simulink model "awe_dt"  (R2024b)
settings: Solver=VariableStepAuto  StartTime=0.0  StopTime=0.001  RelTol=1e-3
model workspace (MAT data in the model file):
  A = Simulink.Parameter
  A.Value = 0.03
  A.Complexity = 'real'
  A.Dimensions = [1 1]
  A.DataType = 'double'
  A.DocUnits = 'm'
  I = Simulink.Parameter
  I.Value = Simulink.data.Expression
  I.Value.ExpressionString = "linspace(0,150,200)"
  I.Complexity = 'real'
  I.Dimensions = -1
  I.DataType = 'auto'
  I.DocUnits = 'A'
  P_an = Simulink.Parameter
  P_an.Value = 1
  P_an.Complexity = 'real'
  P_an.Dimensions = [1 1]
  P_an.DataType = 'auto'
  P_an.DocUnits = 'bar'
  P_cat = Simulink.Parameter
  P_cat.Value = 1
  P_cat.Complexity = 'real'
  P_cat.Dimensions = [1 1]
  P_cat.DataType = 'auto'
  P_cat.DocUnits = 'bar'
  T = Simulink.Parameter
  T.Value = Simulink.data.Expression
  T.Value.ExpressionString = "(linspace(273.15,353.15,8))'"
  T.Complexity = 'real'
  T.Dimensions = -1
  T.DataType = 'auto'
  T.DocUnits = 'K'
  Voltage = Simulink.Signal
  Voltage.Dimensions = -1
  Voltage.DimensionsMode = 'auto'
  Voltage.Complexity = 'auto'
  Voltage.SampleTime = -1
  Voltage.SamplingMode = 'auto'
  Voltage.DataType = 'auto'
  molality_koh = Simulink.Parameter
  molality_koh.Value = 5.94
  molality_koh.Complexity = 'real'
  molality_koh.Dimensions = [1 1]
  molality_koh.DataType = 'auto'
  molality_koh.DocUnits = 'mol/kg'
settings Model: Creator=vr231  LastModifiedBy=jnana

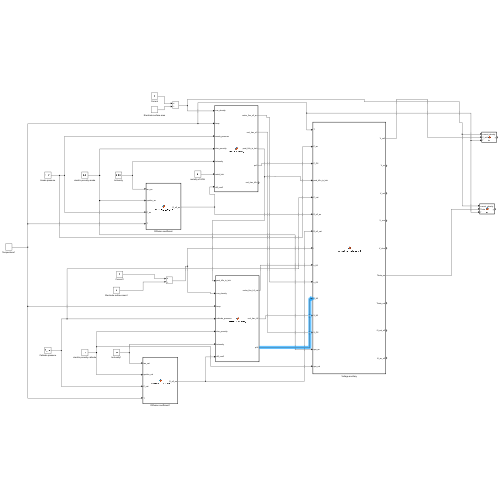
[thumbnail: Simulink's stored preview of the top-level diagram]
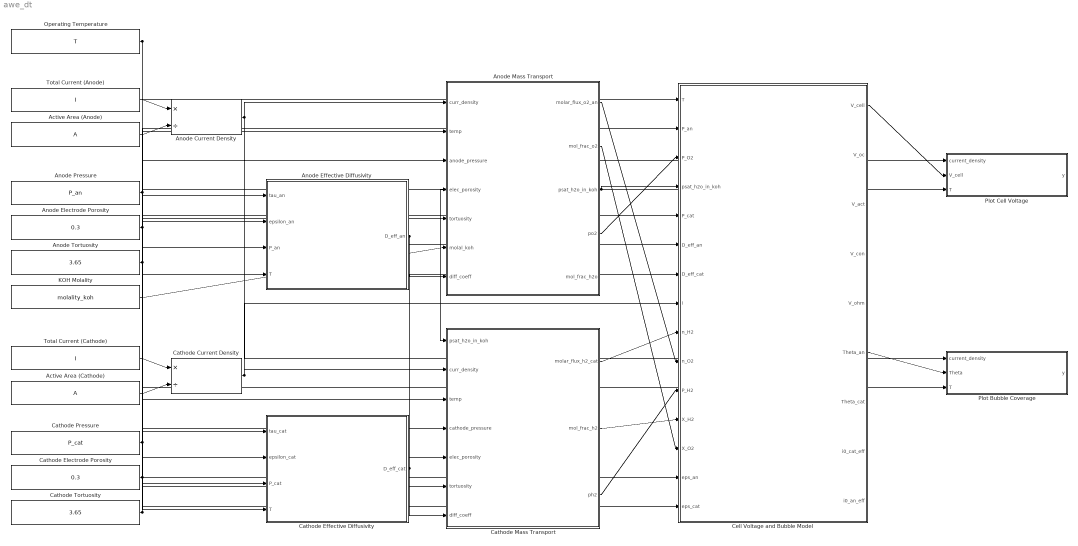
== system awe_dt ==
  Anode Pressure : Constant  Value=P_an
  Cathode Pressure : Constant  Value=P_cat
  Total Current (Anode) : Constant  Value=I
  Total Current (Cathode) : Constant  Value=I
  Anode Effective Diffusivity : MATLAB Function  TreatAsAtomicUnit=on
  Cathode Effective Diffusivity : MATLAB Function  TreatAsAtomicUnit=on
  Anode Current Density : Product  Inputs=*/
  Cathode Current Density : Product  Inputs=*/
  Active Area (Anode) : Constant  Value=A
  Active Area (Cathode) : Constant  Value=A
  Anode Mass Transport : MATLAB Function  TreatAsAtomicUnit=on
  Cathode Mass Transport : MATLAB Function  TreatAsAtomicUnit=on
  Plot Bubble Coverage : MATLAB Function  TreatAsAtomicUnit=on
  Plot Cell Voltage : MATLAB Function  TreatAsAtomicUnit=on
  Operating Temperature : Constant  Value=T
  Cell Voltage and Bubble Model : MATLAB Function  TreatAsAtomicUnit=on
  Anode Electrode Porosity : Constant  Value=0.3
  Cathode Electrode Porosity : Constant  Value=0.3
  KOH Molality : Constant  Value=molality_koh
  Anode Tortuosity : Constant  Value=3.65
  Cathode Tortuosity : Constant  Value=3.65
  wires:
  KOH Molality/1 -> Anode Mass Transport/6(molal_koh)
  Operating Temperature/1 -> Cathode Effective Diffusivity/4(T), Cathode Mass Transport/3(temp), Plot Bubble Coverage/3(T), Plot Cell Voltage/3(T), Cell Voltage and Bubble Model/1(T), Anode Mass Transport/2(temp), Anode Effective Diffusivity/4(T)
  Anode Pressure/1 -> Cell Voltage and Bubble Model/2(P_an), Anode Mass Transport/3(anode_pressure), Anode Effective Diffusivity/3(P_an)
  Total Current (Anode)/1 -> Anode Current Density/1
  Active Area (Anode)/1 -> Anode Current Density/2
  Anode Effective Diffusivity/1(D_eff_an) -> Anode Mass Transport/7(diff_coeff), Cell Voltage and Bubble Model/6(D_eff_an)
  Anode Tortuosity/1 -> Anode Effective Diffusivity/1(tau_an), Anode Mass Transport/5(tortuosity)
  Anode Electrode Porosity/1 -> Cell Voltage and Bubble Model/14(eps_an), Anode Effective Diffusivity/2(epsilon_an), Anode Mass Transport/4(elec_porosity)
  Cathode Effective Diffusivity/1(D_eff_cat) -> Cell Voltage and Bubble Model/7(D_eff_cat), Cathode Mass Transport/7(diff_coeff)
  Cathode Pressure/1 -> Cell Voltage and Bubble Model/5(P_cat), Cathode Mass Transport/4(cathode_pressure), Cathode Effective Diffusivity/3(P_cat)
  Cathode Electrode Porosity/1 -> Cell Voltage and Bubble Model/15(eps_cat), Cathode Mass Transport/5(elec_porosity), Cathode Effective Diffusivity/2(epsilon_cat)
  Active Area (Cathode)/1 -> Cathode Current Density/2
  Cathode Current Density/1 -> Cathode Mass Transport/2(curr_density), Cell Voltage and Bubble Model/8(i)
  Total Current (Cathode)/1 -> Cathode Current Density/1
  Cathode Tortuosity/1 -> Cathode Mass Transport/6(tortuosity), Cathode Effective Diffusivity/1(tau_cat)
  Anode Mass Transport/3(psat_h2o_in_koh) -> Cell Voltage and Bubble Model/4(psat_h2o_in_koh), Cathode Mass Transport/1(psat_h2o_in_koh)
  Anode Mass Transport/1(molar_flux_o2_an) -> Cell Voltage and Bubble Model/10(n_O2)
  Cathode Mass Transport/2(mol_frac_h2) -> Cell Voltage and Bubble Model/12(X_H2)
  Cathode Mass Transport/1(molar_flux_h2_cat) -> Cell Voltage and Bubble Model/9(n_H2)
  Anode Mass Transport/2(mol_frac_o2) -> Cell Voltage and Bubble Model/13(X_O2)
  Cell Voltage and Bubble Model/1(V_cell) -> Plot Cell Voltage/2(V_cell)
  Cathode Mass Transport/3(ph2) -> Cell Voltage and Bubble Model/11(P_H2)
  Cell Voltage and Bubble Model/6(Theta_an) -> Plot Bubble Coverage/2(Theta)
  Anode Current Density/1 -> Plot Bubble Coverage/1(current_density), Plot Cell Voltage/1(current_density), Anode Mass Transport/1(curr_density)
  Anode Mass Transport/4(po2) -> Cell Voltage and Bubble Model/3(P_O2)

== matlab function awe_dt/Plot Bubble Coverage ==
  data: current_density input; y output; Theta input; T input
function y = fcn(current_density, Theta, T)
%#codegen
  % Define graphics functions as extrinsic
  coder.extrinsic('figure','axes','plot','xlabel','ylabel','drawnow','hold','grid','isvalid','cla','box','legend','sprintf');
  
  persistent hFig hAx plot_done
  
  % --- FIGURE SETUP ---
  if isempty(hFig)
      hFig = figure('Name','Theta vs Current','NumberTitle','off');
      hAx  = axes('Parent',hFig);
      xlabel(hAx,'Current Density (A/m^2)');  
      ylabel(hAx,'Bubble Coverage (Theta)');
      grid(hAx, 'on'); box(hAx, 'on'); hold(hAx, 'on');
      plot_done = [];
  end
  
  if ~isvalid(hFig)
      hFig = figure('Name','Theta vs Current','NumberTitle','off');
      hAx  = axes('Parent',hFig);
      xlabel(hAx,'Current Density (A/m^2)');  
      ylabel(hAx,'Bubble Coverage (Theta)');
      grid(hAx, 'on'); box(hAx, 'on'); hold(hAx, 'on');
      plot_done = [];
  end
  
  % --- DATA PREP (No Resizing Inputs) ---
  u_plot = double(current_density); 
  v_plot = double(Theta);           
  T_vals = double(T);            
  
  % Transpose logic for PLOTTING ONLY. 
  if size(v_plot, 2) == numel(u_plot)
      v_plot_T = v_plot.'; 
  else
      v_plot_T = v_plot;
  end
  
  % --- PLOT ---
  if isempty(plot_done)
      cla(hAx); 
      plot(hAx, u_plot, v_plot_T, '-o', 'LineWidth', 1.5, 'MarkerSize', 4);
      
      % --- LEGEND (Extrinsic Call) ---
      update_legend(hAx, T_vals);
      
      drawnow;
      plot_done = 1;
  end
  % --- OUTPUT ---
  y = Theta;
end

% --- SUB-FUNCTION (Runs in MATLAB only) ---
function update_legend(ax_handle, T_vals)
    if numel(T_vals) > 0
        labels = cell(1, numel(T_vals));
        for k = 1:numel(T_vals)
            % CHANGED: Using sprintf instead of num2str
            labels{k} = sprintf('T = %.1f K', T_vals(k));
        end
        legend(ax_handle, labels, 'Location', 'best');
    end
end

== matlab function awe_dt/Plot Cell Voltage ==
  data: current_density input; y output; V_cell input; T input
function y = fcn(current_density, V_cell, T)
%#codegen
  % Define graphics functions as extrinsic
  coder.extrinsic('figure','axes','plot','xlabel','ylabel','drawnow','hold','grid','isvalid','cla','box','legend','sprintf');
  
  persistent hFig hAx plot_done
  
  % --- FIGURE SETUP ---
  if isempty(hFig)
      hFig = figure('Name','Voltage vs Current','NumberTitle','off');
      hAx  = axes('Parent',hFig);
      xlabel(hAx,'Current Density (A/m^2)');  
      ylabel(hAx,'Cell Voltage (V)');
      grid(hAx, 'on'); box(hAx, 'on'); hold(hAx, 'on');    
      plot_done = [];
  end
  
  if ~isvalid(hFig)
      hFig = figure('Name','Voltage vs Current','NumberTitle','off');
      hAx  = axes('Parent',hFig);
      xlabel(hAx,'Current Density (A/m^2)');  
      ylabel(hAx,'Cell Voltage (V)');
      grid(hAx, 'on'); box(hAx, 'on'); hold(hAx, 'on');
      plot_done = [];
  end
  
  % --- DATA PREP (No Resizing Inputs) ---
  if isempty(plot_done)
      u_plot = double(current_density); 
      v_plot = double(V_cell);           
      T_vals = double(T);            
      
      % Transpose logic for PLOTTING ONLY. 
      % We assume u_plot is 1x201. v_plot is 8x201.
      % Plot expects 201x8.
      if size(v_plot, 2) == numel(u_plot)
          v_plot_T = v_plot.'; 
      else
          v_plot_T = v_plot;
      end
      
      % --- PLOT ---
      cla(hAx); 
      plot(hAx, u_plot, v_plot_T, 'o', 'LineWidth', 1.5, 'MarkerSize', 4);
      
      % --- LEGEND (Extrinsic Call) ---
      update_legend(hAx, T_vals);
      
      drawnow;
      plot_done = 1;
  end 
  % --- OUTPUT ---
  y = V_cell;
end

% --- SUB-FUNCTION (Runs in MATLAB only) ---
function update_legend(ax_handle, T_vals)
    if numel(T_vals) > 0
        labels = cell(1, numel(T_vals));
        for k = 1:numel(T_vals)
            % Clean formatting for Legend
            labels{k} = sprintf('T = %.1f K', T_vals(k));
        end
        legend(ax_handle, labels, 'Location', 'best');
    end
end

== matlab function awe_dt/Anode Effective Diffusivity ==
  data: tau_an input; epsilon_an input; P_an input; T input; D_eff_an output
function D_eff_an = calculate_D_eff_an( tau_an,epsilon_an,P_an,T)
    % Calculates the effective binary diffusion coefficient at the anode (D_eff_an)
    % according to equations 38-46 from Abdin et al. (2017)
    %
    % Inputs:
    %   T - Temperature [K]
    %   P_an - Anode pressure [Pa]
    %   epsilon_an - Anode porosity [dimensionless]
    %   tau_an - Anode tortuosity [dimensionless]
    %
    % Output:
    %   D_eff_an - Effective binary diffusion coefficient at anode [m^2/s]

    % Constants
    R = 8.314;               % Universal gas constant [J/(mol·K)]
    k = 1.38064852e-23;      % Boltzmann constant [J/K]
    
    % Molecular weights [kg/mol]
    M_O2 = 32e-3;
    M_H2O = 18e-3;
    
    % Molecular radii [m] (converted from Å)
    sigma_O2 = 3.467e-10;
    sigma_H2O = 2.641e-10;
    
    % Lennard-Jones potentials [K]
    epsilon_O2_k = 106.7;    % epsilon/k for O2
    epsilon_H2O_k = 809.1;   % epsilon/k for H2O
    
    % Convert Lennard-Jones potentials to Joules
    epsilon_O2 = epsilon_O2_k * k;
    epsilon_H2O = epsilon_H2O_k * k;
    
    % Mean pore radius [m] (typical value, can be adjusted)
    r = 75e-9;                % 75 nm
    
    % Calculate mean molecular radius (Eq. 44)
    sigma_O2_H2O = (sigma_O2 + sigma_H2O)/2;
    
    % Calculate Lennard-Jones energy (Eq. 46)
    epsilon_O2_H2O = sqrt(epsilon_O2 * epsilon_H2O);
    
    % Calculate reduced temperature (Eq. 45)
    tau_O2_H2O = k .* T / epsilon_O2_H2O;
    
    % Calculate dimensionless diffusion collision integral (Eq. 43)
    Omega_D = 1.06./(tau_O2_H2O.^0.156) + 0.193./exp(0.476.*tau_O2_H2O) + ...
              1.036./exp(1.53.*tau_O2_H2O) + 1.765./(3.894.*tau_O2_H2O);
    
    % Calculate effective molecular binary diffusion coefficient (Eq. 41)
    D_eff_O2_H2O = 0.00133 .* (1/M_O2 + 1/M_H2O)^0.5 .* T.^1.5 ./ ...
                  (P_an.*(10^5).* sigma_O2_H2O^2 .* Omega_D);
    
    % Calculate effective Knudsen diffusion coefficient (Eq. 40)
    D_eff_H2O_K = (4/3) * r * sqrt((8 * R .* T) / (pi * M_H2O));
    
    % Calculate effective binary diffusion coefficient at anode (Eq. 38)
    D_eff_an = ((epsilon_an ./ tau_an) .* (1./D_eff_O2_H2O + 1./D_eff_H2O_K).^-1);
end

== matlab function awe_dt/Anode Mass Transport ==
  data: curr_density input; temp input; molar_flux_o2_an output; anode_pressure input; elec_porosity input; mol_frac_o2 output; psat_h2o_in_koh output; po2 output; tortuosity input; molal_koh input; diff_coeff input; mol_frac_h2o output
function [molar_flux_o2_an, mol_frac_o2, psat_h2o_in_koh, po2, mol_frac_h2o] = anode_ancillary(curr_density, temp, anode_pressure, elec_porosity, tortuosity, molal_koh, diff_coeff)
    % Constants
    faraday_const = 96485;       % C/mol
    univ_gas_const = 8.314;       % J/(mol·K)
    len_an_to_catalyst = 0.002;   % m

    % Ensure vector orientations
    curr_density = curr_density(:).';  % Force row vector [1×m]
    temp = temp(:);                    % Force column vector [n×1]
    
    % Nested function for water vapor pressure
    function log_pw = calculate_logpw(m, T)
        term1 = -0.01508*m - 0.0016788*m.^2 + 2.25887e-5*m.^3;
        poly_m = 1 - 0.0012062*m + 5.6024e-4*m.^2 - 7.8228e-6*m.^3;
        term_T = 35.4462 - 3343.93./T - 10.9*log10(T) + 0.0041645*T;
        log_pw = term1 + poly_m.*term_T;
    end

    % 1. Calculate water vapor pressure [n×1]
    psat_h2o_in_koh = 10.^(calculate_logpw(molal_koh, temp));  % bar

    % 2. Molar oxygen flux [1×m]
    molar_flux_o2_an = curr_density ./ (4 * faraday_const);  % mol/(m²·s)

    % 3. Water mole fraction calculation [n×m]
    R = univ_gas_const;
    L = len_an_to_catalyst;
    F = faraday_const;
    P = anode_pressure * 1e5;  % Convert bar to Pa
    
    % Calculate exponent term with dimensional consistency
    exponent_term = (R * L) ./ (2 * F * P * diff_coeff) .* (curr_density .* temp);
    
    % Clamp exponent to prevent overflow
    max_exp = 700;  % exp(700) ≈ 1e304 (below realmax)
    exponent_term = min(exponent_term, max_exp);
    
    % Calculate mole fraction with safeguards
    mol_frac_h2o = (elec_porosity/tortuosity) .* exp(exponent_term);
    mol_frac_h2o = min(mol_frac_h2o, 1);  % Prevent values >1
    mol_frac_h2o = max(mol_frac_h2o, 0);  % Prevent negative values

    % 4. Oxygen mole fraction [n×m]
    mol_frac_o2 = 1 - mol_frac_h2o;

    % 5. Oxygen partial pressure [n×m]
    po2 = ((1 ./ mol_frac_h2o) - 1) .* psat_h2o_in_koh;  % bar
end

== matlab function awe_dt/Cathode Effective Diffusivity ==
  data: tau_cat input; epsilon_cat input; P_cat input; T input; D_eff_cat output
function D_eff_cat = calculate_D_eff_cat( tau_cat,epsilon_cat,P_cat,T)
    % Calculates the effective binary diffusion coefficient at the anode (D_eff_cat)
    % according to equations 38-46 from Abdin et al. (2017)
    %
    % Inputs:
    %   T - Temperature [K]
    %   P_an - Anode pressure [Pa]
    %   epsilon_an - Anode porosity [dimensionless]
    %   tau_an - Anode tortuosity [dimensionless]
    %
    % Output:
    %   D_eff_cat - Effective binary diffusion coefficient at anode [m^2/s]

    % Constants
    R = 8.314;               % Universal gas constant [J/(mol·K)]
    k = 1.38064852e-23;      % Boltzmann constant [J/K]
    
    % Molecular weights [kg/mol]
    M_O2 = 32e-3;
    M_H2O = 18e-3;
    
    % Molecular radii [m] (converted from Å)
    sigma_O2 = 3.467e-10;
    sigma_H2O = 2.641e-10;
    
    % Lennard-Jones potentials [K]
    epsilon_O2_k = 106.7;    % epsilon/k for O2
    epsilon_H2O_k = 809.1;   % epsilon/k for H2O
    
    % Convert Lennard-Jones potentials to Joules
    epsilon_O2 = epsilon_O2_k * k;
    epsilon_H2O = epsilon_H2O_k * k;
    
    % Mean pore radius [m] (typical value, can be adjusted)
    r = 75e-9;                % 75 nm
    
    % Calculate mean molecular radius (Eq. 44)
    sigma_O2_H2O = (sigma_O2 + sigma_H2O)/2;
    
    % Calculate Lennard-Jones energy (Eq. 46)
    epsilon_O2_H2O = sqrt(epsilon_O2 * epsilon_H2O);
    
    % Calculate reduced temperature (Eq. 45)
    tau_O2_H2O = k .* T / epsilon_O2_H2O;
    
    % Calculate dimensionless diffusion collision integral (Eq. 43)
    Omega_D = 1.06./(tau_O2_H2O.^0.156) + 0.193./exp(0.476.*tau_O2_H2O) + ...
              1.036./exp(1.53.*tau_O2_H2O) + 1.765./(3.894.*tau_O2_H2O);
    
    % Calculate effective molecular binary diffusion coefficient (Eq. 41)
    D_eff_O2_H2O = 0.00133 .* (1/M_O2 + 1/M_H2O)^0.5 .* T.^1.5 ./ ...
                  (P_cat.*(10^5).* sigma_O2_H2O^2 .* Omega_D);
    
    % Calculate effective Knudsen diffusion coefficient (Eq. 40)
    D_eff_H2O_K = (4/3) * r * sqrt((8 * R .* T) / (pi * M_H2O));
    
    % Calculate effective binary diffusion coefficient at anode (Eq. 38)
    D_eff_cat = ((epsilon_cat ./ tau_cat) .* (1./D_eff_O2_H2O + 1./D_eff_H2O_K).^-1);
end

== matlab function awe_dt/Cathode Mass Transport ==
  data: psat_h2o_in_koh input; curr_density input; temp input; cathode_pressure input; molar_flux_h2_cat output; elec_porosity input; mol_frac_h2 output; ph2 output; tortuosity input; diff_coeff input
function [molar_flux_h2_cat, mol_frac_h2, ph2] = cathode_ancillary(psat_h2o_in_koh, curr_density, temp, cathode_pressure, elec_porosity, tortuosity, diff_coeff)
    % Constants
    faraday_const = 96485;       % C/mol
    univ_gas_const = 8.314;      % J/(mol·K)
    len_catalyst_to_cat = 0.002; % m
    
    % Force vector orientations
    curr_density = curr_density(:).';  % Row vector [1×m]
    temp = temp(:);                    % Column vector [n×1]
    
    % 1. Molar hydrogen flux [m×1]
    molar_flux_h2_cat = (curr_density ./ (2 * faraday_const))';
    
    % 2. Water mole fraction calculation [n×m]
    R = univ_gas_const;
    L = len_catalyst_to_cat;
    F = faraday_const;
    P = cathode_pressure * 1e5;  % Convert bar to Pa
    
    % Calculate exponent term with proper broadcasting
    exponent_term = (R * L) ./ (2 * F * P * diff_coeff) .* (curr_density .* temp);
    
    % Clamp exponent to prevent overflow
    max_exp = 700;  % exp(700) ≈ 1e304 (below realmax)
    exponent_term = min(exponent_term, max_exp);
    
    % Calculate mole fraction with safeguards
    mol_frac_h20 = (elec_porosity/tortuosity) .* exp(exponent_term);
    mol_frac_h20 = min(mol_frac_h20, 1);  % Prevent >100% coverage
    mol_frac_h20 = max(mol_frac_h20, 0);  % Prevent negative values
    
    % 3. Hydrogen mole fraction [n×m]
    mol_frac_h2 = 1 - mol_frac_h20;
    
    % 4. Hydrogen partial pressure [n×m]
    ph2 = ((1 ./ mol_frac_h20) - 1) .* psat_h2o_in_koh;  % bar
end

== matlab function awe_dt/Cell Voltage and Bubble Model ==
  data: T input; V_cell output; P_an input; P_O2 input; psat_h2o_in_koh input; P_cat input; D_eff_an input; D_eff_cat input; i input; n_H2 input; n_O2 input; P_H2 input; X_H2 input; X_O2 input; eps_an input; eps_cat input; V_oc output; V_act output; V_con output; V_ohm output; Theta_an output; Theta_cat output; i0_cat_eff output; i0_an_eff output

function [V_cell, V_oc,V_act,V_con,V_ohm, Theta_an, Theta_cat, i0_cat_eff, i0_an_eff] = electrolyser_voltage_nd(...
    T, P_an,P_O2,psat_h2o_in_koh, P_cat, D_eff_an, D_eff_cat, i, n_H2, n_O2,P_H2, X_H2, X_O2, eps_an, eps_cat)
% Vectorized alkaline electrolyser voltage model for N-D arrays
% Inputs and constants unchanged; only V_components packaging updated

%% Constants and parameters
F      = 96485;      R      = 8.314;    T_ref  = 298.15;     V_std0 = 1.229;
params.gamma_M_an = 1.25; params.gamma_M_cat = 1.05;
params.DG_c_an = 80e3;    params.DG_c_cat = 51e3;
params.i0_an_ref = 1e-7;   params.i0_cat_ref = 10;
params.alpha_an = 1.65;   params.alpha_cat = 0.73;
params.delta_an = 0.002;  params.delta_cat = 0.002; params.A_e = 0.03;
params.l_an_s = 0.00125;  params.l_cat_s = 0.00125;
params.beta_an = 0.00045; params.beta_cat = 0.00045;
params.rho_el_ref = 0.00167; params.kappa_el = -0.02;
params.delta_s = 0.0005;  params.epsilon_s = 0.42;
params.tau_s = 2.18;      params.omega_s = 0.85; params.A_s = 0.03;
params.rho_an = 1e-6;     params.rho_cat = 1e-6;
params.kappa_an = 0.003;  params.kappa_cat = 0.003;
%% 1. Open-circuit voltage

a_H2O_KOH = 0.82; % deltaS0byNf equals -0.9e-3

% Ensure proper dimensions for broadcasting
T = T(:);           % Force [2x1] column vector
i = i(:)';          % Force [1x201] row vector
% Inputs:
% T = [2x1] column vector (temperatures)
% i = [1x201] row vector (current densities)
% P_H2, P_O2 = scalar or [1x201] (pressure terms, adjust as needed)

% Ensure T is column vector and i is row vector
T = T(:);  % [2x1]
i = i(:).'; % [1x201]

% Calculate V_oc with proper broadcasting
log_term = log( (P_H2 .* sqrt(P_O2)) ./ a_H2O_KOH ); % Scalar or [1x201]

V_oc = V_std0 + ...
       (T - T_ref) .* (-0.9e-3) + ...  % [2x1]
       (R .* T / (2*F)) .* log_term;           % [2x1] or [2x201]

% Explicitly expand V_oc to [2x201] if log_term is scalar
if isscalar(log_term)
    V_oc = V_oc1 .* ones(1, numel(i));  % [2x1] => [2x201]
end


%% 2. Activation overpotential
i_lim = 30e3;
%Bubble Coverage: Viscosity-Based Arrhenius Model
% ---------------------------------------------------------
% Instead of the Abdin polynomial (which fails at low T), we scale 
% coverage based on the exponential decay of electrolyte viscosity.
% Ref: Analogous to Vogel-Fulcher-Tammann or Arrhenius viscosity laws
% "Activation Energy" for Bubble Detachment
% A value of ~1500-2500 mimics the drop in water viscosity from 25C to 80C.
% You can tune this 'B_visc' value:
% Higher (e.g., 3000) = Bubbles drop off VERY fast as it heats up.
% Lower (e.g., 1000) = Bubbles stick longer.
B_visc = 2000;
temp_coeff = exp(B_visc*((1./T) - (1./T_ref)));  % [2x1]
current_coeff = (i./i_lim).^0.3;                            % [1x201]
pressure_term_an = P_an./(P_an - psat_h2o_in_koh);         % [2x1]
pressure_term_cat = P_cat./(P_cat - psat_h2o_in_koh);      % [2x1]
% Base Coverage Factor (Tuned to match ~0.15 - 0.2 at standard conditions)
theta_base = 0.5;
Theta_an = theta_base.* temp_coeff .* current_coeff .* pressure_term_an;   % [2x201] via broadcasting
Theta_cat = theta_base.* temp_coeff .* current_coeff .* pressure_term_cat; % [2x201] via broadcasting

Theta_an  = min(max(Theta_an, 1e-6), 0.99);
Theta_cat = min(max(Theta_cat, 1e-6), 0.99);

% Exchange current densities
i0_an_eff = params.gamma_M_an .* exp(-params.DG_c_an./R .* (1./T - 1./T_ref)) .* params.i0_an_ref;  % [2x1]
i0_cat_eff = params.gamma_M_cat .* exp(-params.DG_c_cat./R .* (1./T - 1./T_ref)) .* params.i0_cat_ref; % [2x1]

% Activation overpotentials with proper broadcasting
V_act_an = ((R.*T./(params.alpha_an*F)) .* log(i./(i0_an_eff))).*(1+(0.2.*((T./T_ref).^4)).*current_coeff.* pressure_term_an); % [2x201]
V_act_cat = ((R.*T./(params.alpha_cat*F)) .* log(i./(i0_cat_eff))).*(1+(0.2.*((T./T_ref).^4)).*current_coeff.* pressure_term_cat); % [2x201]
V_act = V_act_an + V_act_cat; % [2x201]

%% 3. Concentration overpotential
C_O2_0 = P_an.*(10^5).*X_O2./(R.*T);  % [2x201] (assuming X_O2 is [2x201])
C_H2_0 = P_cat.*(10^5).*X_H2./(R.*T); % [2x201] (assuming X_H2 is [2x201])

% Ensure n_O2 and n_H2 have compatible dimensions for broadcasting
C_O2_el = C_O2_0 + (params.delta_an./D_eff_an) .* n_O2; % [2x201]
C_H2_el = C_H2_0 + (params.delta_cat./D_eff_cat) .* (n_H2)'; % [2x201]

V_con = (R.*T./(4*F)).*log(C_O2_el./C_O2_0) + (R.*T./(2*F)).*log(C_H2_el./C_H2_0); % [2x201]

%% 4. Ohmic overpotential
% -- Electrolyte Resistivity (Gilliam et al. 2007 approx for 30wt% KOH) --
% This replaces the broken linear model. 
% If you want to use your params.rho_el_ref, use an exponential decay:
% rho_el = params.rho_el_ref .* exp( -0.015 .* (T - T_ref) ); 

% Or using a high-fidelity correlation (Recommended for Digital Twin):
% Molarity of 30wt% KOH ~ 6.9 M
M = 6.9; 
T_C = T - 273.15;
sigma_KOH = ( -2.041*M - 0.0028*M^2 + 0.005332*M*T_C + 20.72*T_C/T_ref ) * 10; % Rough approx
% Arrhenius scaling creates a massive drop in resistance as T rises
rho_el = params.rho_el_ref .* exp( (15000/R) .* (1./T - 1./T_ref) );
% Simplified safe fallback for your specific structure:
%rho_el = 0.01 ./ (0.5 + 0.015 * (T - 273.15)); % Ensures positive
%resistivity (linear model, can be incorrect)

% -- Electrode Resistances --
% Using exponential term for temperature dependence of metal resistivity to be safe
alpha_metal = 0.003; % Typical coeff for metals
R_an = params.rho_an ./ (1-eps_an).^1.5 .* params.delta_an./params.A_e .* (1 + alpha_metal.*(T-T_ref));
R_cat = params.rho_cat ./ (1-eps_cat).^1.5 .* params.delta_cat./params.A_e .* (1 + alpha_metal.*(T-T_ref));
R_electrodes = R_an + R_cat;
% -- Bubble Resistance (Bruggeman) --
R_el_an = rho_el .* ((params.l_an_s - params.beta_an)./params.A_e + ...
          params.beta_an ./ (params.A_e .* (1-Theta_an).^1.5));
      
R_el_cat = rho_el .* ((params.l_cat_s - params.beta_cat)./params.A_e + ...
           params.beta_cat ./ (params.A_e .* (1-Theta_cat).^1.5));
       
R_el = R_el_an + R_el_cat;

% -- Separator Resistance --
R_s = rho_el .* params.tau_s.^2 .* params.delta_s ./ (params.omega_s .* params.epsilon_s .* params.A_s);

% Total Ohmic
I_matrix = i * params.A_e; % Convert current density to current and ensure [1x201]
V_ohm = I_matrix .* (R_electrodes + R_el + R_s);

%% 5. Total cell voltage
V_cell = V_oc + V_act + V_con + V_ohm; % All [2x201]
% Zero current cleanup
zero_idx = abs(i) < 1e-6;
if any(zero_idx)
     % Force total voltage to Open Circuit Voltage (OCV)
     % This implicitly means V_act, V_con, V_ohm are all 0.
     V_cell(:, zero_idx) = V_oc(:, zero_idx);
end
